simulink model "basic_model_4x2"  (R2023b)
settings: Solver=VariableStepAuto  StartTime=0.0  StopTime=150  RelTol=1e-3
undefined symbols (not defined in the file): ac, sys_mimo_2x2, sys_mimo_4x2
libraries: simulink x2
settings Model: Creator=kaleb  LastModifiedBy=kaleb

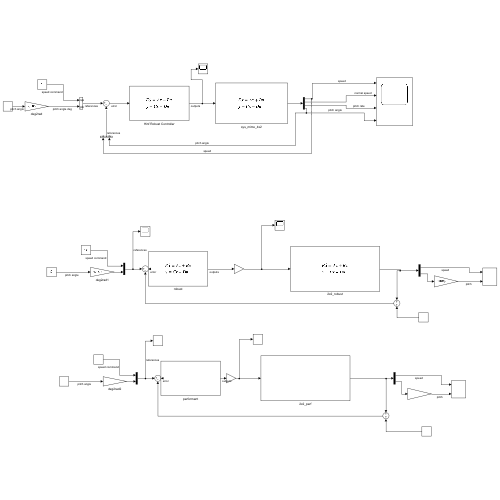
[thumbnail: Simulink's stored preview of the top-level diagram]
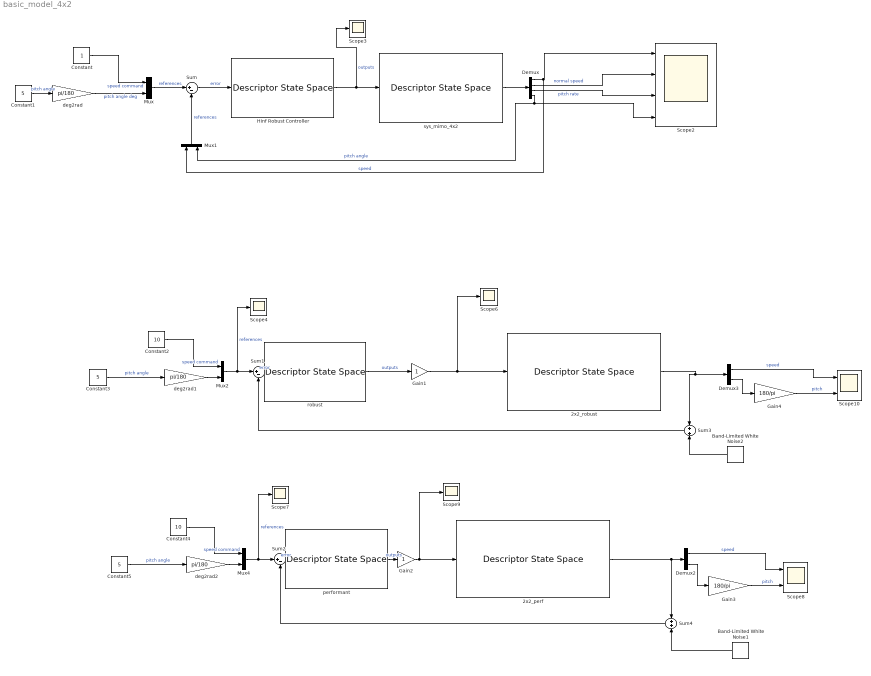
== system basic_model_4x2 ==
  2x2_perf : DescriptorStateSpace  E=eye(2)  A=sys_mimo_2x2.A  B=sys_mimo_2x2.B  C=sys_mimo_2x2.C  D=sys_mimo_2x2.D  InitialCondition=[0,0]  DirectFeedthrough=False
  2x2_robust : DescriptorStateSpace  E=eye(2)  A=sys_mimo_2x2.A  B=sys_mimo_2x2.B  C=sys_mimo_2x2.C  D=sys_mimo_2x2.D  InitialCondition=[0,0]  DirectFeedthrough=False
  Band-Limited White Noise1 : simulink/Sources/Band-Limited White Noise  Cov=[0.5, 0.05/50]  Ts=0.1  seed=[23341]
  Band-Limited White Noise2 : simulink/Sources/Band-Limited White Noise  Cov=[0.5, 0.05/50]  Ts=0.1  seed=[23341]
  Constant : Constant
  Constant1 : Constant  Value=5
  Constant2 : Constant  Value=10
  Constant3 : Constant  Value=5
  Constant4 : Constant  Value=10
  Constant5 : Constant  Value=5
  Demux : Demux
  Demux2 : Demux  Outputs=2
  Demux3 : Demux  Outputs=2
  Gain1 : Gain
  Gain2 : Gain
  Gain3 : Gain  Gain=180/pi
  Gain4 : Gain  Gain=180/pi
  Hinf Robust Controller : DescriptorStateSpace  E=eye(6)  A=ac.ltf_robust.Gc.A  B=ac.ltf_robust.Gc.B  C=ac.ltf_robust.Gc.C  D=ac.ltf_robust.Gc.D  InitialCondition=[0,0, 0,0,0,0]  DirectFeedthrough=False
  Mux{,1..2,4} (4 alike) : Mux  Inputs=2
      Mux settings: DisplayOption=signals
      Mux1 settings: DisplayOption=signals
  Scope10 : Scope  NumInputPorts=2
  Scope2 : Scope  NumInputPorts=4
  Scope{3..4,6..7,9} (5 alike) : Scope
  Scope8 : Scope  NumInputPorts=2
  Sum : Sum  Inputs=|+-
  Sum1 : Sum  Inputs=|+-
  Sum2 : Sum  Inputs=|+-
  Sum3 : Sum  Inputs=+|+
  Sum4 : Sum  Inputs=+|+
  deg2rad : Gain  Gain=pi/180
  deg2rad1 : Gain  Gain=pi/180
  deg2rad2 : Gain  Gain=pi/180
  performant : DescriptorStateSpace  E=eye(6)  A=ac.ltf_performant.Gc.A  B=ac.ltf_performant.Gc.B  C=ac.ltf_performant.Gc.C  D=ac.ltf_performant.Gc.D  InitialCondition=[0,0, 0,0,0,0]  DirectFeedthrough=False
  robust : DescriptorStateSpace  E=eye(6)  A=ac.ltf_robust.Gc.A  B=ac.ltf_robust.Gc.B  C=ac.ltf_robust.Gc.C  D=ac.ltf_robust.Gc.D  InitialCondition=[0,0, 0,0,0,0]  DirectFeedthrough=False
  sys_mimo_4x2 : DescriptorStateSpace  E=eye(4)  A=sys_mimo_4x2.A  B=sys_mimo_4x2.B  C=sys_mimo_4x2.C  D=sys_mimo_4x2.D  InitialCondition=[0,0,0, 0]  DirectFeedthrough=False
  wires:
  Constant1/1 -> deg2rad/1  "pitch angle"
  Constant/1 -> Mux/1  "speed command"
  Mux/1 -> Sum/1  "references"
  deg2rad/1 -> Mux/2  "pitch angle deg"
  sys_mimo_4x2/1 -> Demux/1
  Demux/1 -> Mux1/1, Scope2/1  "speed"
  Gain1/1 -> Scope6/1, 2x2_robust/1
  Mux2/1 -> Scope4/1, Sum1/1  "references"
  Sum1/1 -> robust/1  "error"
  robust/1 -> Gain1/1  "outputs"
  deg2rad1/1 -> Mux2/2
  Constant3/1 -> deg2rad1/1  "pitch angle"
  Constant2/1 -> Mux2/1  "speed command"
  2x2_robust/1 -> Sum3/1, Demux3/1
  Hinf Robust Controller/1 -> Scope3/1, sys_mimo_4x2/1  "outputs"
  Sum2/1 -> performant/1  "error"
  Constant5/1 -> deg2rad2/1  "pitch angle"
  Mux4/1 -> Scope7/1, Sum2/1  "references"
  performant/1 -> Gain2/1  "outputs"
  2x2_perf/1 -> Demux2/1, Sum4/1
  deg2rad2/1 -> Mux4/2
  Constant4/1 -> Mux4/1  "speed command"
  Gain2/1 -> Scope9/1, 2x2_perf/1
  Demux2/1 -> Scope8/1  "speed"
  Demux2/2 -> Gain3/1
  Gain3/1 -> Scope8/2  "pitch"
  Demux3/2 -> Gain4/1
  Gain4/1 -> Scope10/2  "pitch"
  Demux3/1 -> Scope10/1  "speed"
  Sum3/1 -> Sum1/2
  Band-Limited White Noise1/1 -> Sum4/2
  Sum4/1 -> Sum2/2
  Band-Limited White Noise2/1 -> Sum3/2
  Demux/4 -> Scope2/4, Mux1/2  "pitch angle"
  Demux/2 -> Scope2/2  "normal speed"
  Demux/3 -> Scope2/3  "pitch rate"
  Mux1/1 -> Sum/2  "references"
  Sum/1 -> Hinf Robust Controller/1  "error"
